simulink model "2014_BEST_default_v5_simulink"  (R2014a)
settings: Solver=FixedStepDiscrete  StartTime=0.0  StopTime=inf  RelTol=1e-3
libraries: vexarmcortexlib x47, simulink x4
settings Model: Creator=shiremat  LastModifiedBy=Caleb Walke
settings DataIOCC: SignalLoggingSaveFormat=ModelDataLogs
settings OptimizationCC: ExpressionDepthLimit=2147483647  OptimizeModelRefInitCode=on  LifeSpan=Inf  MaxStackSize=64
settings DebuggingCC: UnderspecifiedInitializationDetection=Classic  SolverPrmCheckMsg=none  InheritedTsInSrcMsg=none  ParameterPrecisionLossMsg=none  FcnCallInpInsideContextMsg=UseLocalSettings  UnconnectedInputMsg=none  UnconnectedOutputMsg=none  StateNameClashWarn=warning
settings HardwareCC: ProdLargestAtomicInteger=Long  ProdLargestAtomicFloat=Double  ProdIntDivRoundTo=Floor  ProdEndianess=LittleEndian  ProdHWDeviceType=ARM Compatible->ARM Cortex
settings RTWCC: SystemTargetFile=ert.tlc  TemplateMakefile=ert_default_tmf  Description=Embedded Coder  ProcessScript=ert_make_rtw_hook  Toolchain=GNU Tools for VEX ARM Cortex
settings CodeAppCC: IgnoreCustomStorageClasses=off  CustomSymbolStrType=$N$R$M  InternalIdentifier=Classic
settings ERTTargetCC: CodeReplacementLibrary=GCC ARM Cortex-M3  ParMdlRefBuildCompliant=on  CompOptLevelCompliant=on  ConcurrentExecutionCompliant=on  ERTFirstTimeCompliant=on  ModelStepFunctionPrototypeControlCompliant=on  CPPClassGenCompliant=on  InlinedParameterPlacement=Hierarchical

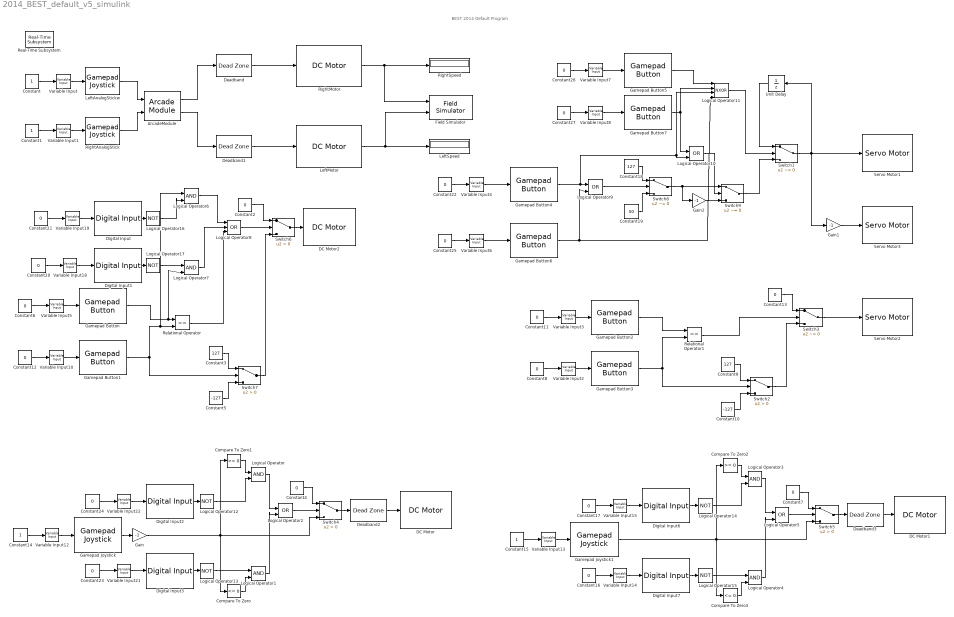
== system 2014_BEST_default_v5_simulink ==
  note: BEST 2014 Default Program
  ArcadeModule : vexarmcortexlib/Utilities/Arcade Module
  Compare To Zero : simulink/Logic and Bit Operations/Compare To Zero  relop=<=  OutDataTypeStr=boolean
  Compare To Zero1 : simulink/Logic and Bit Operations/Compare To Zero  relop=>=  OutDataTypeStr=boolean
  Compare To Zero2 : simulink/Logic and Bit Operations/Compare To Zero  relop=>=  OutDataTypeStr=boolean
  Compare To Zero3 : simulink/Logic and Bit Operations/Compare To Zero  relop=<=  OutDataTypeStr=boolean
  Constant{,1,14..15} (4 alike) : Constant
  Constant10 : Constant  Value=-127
  Constant{6,8,11..13,16..17,20..27} (15 alike) : Constant  Value=0  OutDataTypeStr=boolean
  Constant18 : Constant  Value=127
  Constant19 : Constant  Value=50
  Constant2 : Constant  Value=0
  Constant3 : Constant  Value=127
  Constant4 : Constant  Value=0
  Constant5 : Constant  Value=-127
  Constant7 : Constant  Value=0
  Constant9 : Constant  Value=127
  DC Motor : vexarmcortexlib/DC Motor  motor=5  scaleFactor=1/13.5
  DC Motor1 : vexarmcortexlib/DC Motor  motor=6  scaleFactor=1/13.5
  DC Motor2 : vexarmcortexlib/DC Motor  motor=3  scaleFactor=1/13.5
  Deadband{,1..3} (4 alike) : DeadZone  LowerValue=-4  UpperValue=4  SaturateOnIntegerOverflow=on
  Digital Input : vexarmcortexlib/Digital Input  inChan=1
  Digital Input1 : vexarmcortexlib/Digital Input  inChan=2
  Digital Input2 : vexarmcortexlib/Digital Input  inChan=3
  Digital Input3 : vexarmcortexlib/Digital Input  inChan=4
  Digital Input6 : vexarmcortexlib/Digital Input  inChan=5
  Digital Input7 : vexarmcortexlib/Digital Input  inChan=6
  Field Simulator : vexarmcortexlib/Utilities/Field Simulator  radius=2.5  space=10  range=200
  Gain : Gain  Gain=-1  OutDataTypeStr=Inherit: Inherit via back propagation
  Gain1 : Gain  Gain=-1
  Gain2 : Gain  Gain=-1
  Gamepad Button : vexarmcortexlib/Gamepad Button  joystick=1  chan=5  button56=Down  button78=Right
  Gamepad Button1 : vexarmcortexlib/Gamepad Button  joystick=1  chan=5  button56=Up  button78=Right
  Gamepad Button2 : vexarmcortexlib/Gamepad Button  joystick=1  chan=6  button56=Down  button78=Right
  Gamepad Button3 : vexarmcortexlib/Gamepad Button  joystick=1  chan=6  button56=Up  button78=Right
  Gamepad Button4 : vexarmcortexlib/Gamepad Button  joystick=1  chan=7  button56=Down  button78=Left
  Gamepad Button5 : vexarmcortexlib/Gamepad Button  joystick=1  chan=7  button56=Down  button78=Right
  Gamepad Button6 : vexarmcortexlib/Gamepad Button  joystick=1  chan=7  button56=Down  button78=Down
  Gamepad Button7 : vexarmcortexlib/Gamepad Button  joystick=1  chan=7  button56=Down  button78=Up
  Gamepad Joystick : vexarmcortexlib/Gamepad Joystick  joystick=1  chan=3
  Gamepad Joystick1 : vexarmcortexlib/Gamepad Joystick  joystick=1  chan=4
  LeftAnalogStickw : vexarmcortexlib/Gamepad Joystick  joystick=1  chan=2
  LeftMotor : vexarmcortexlib/DC Motor  motor=9  scaleFactor=1/13.5
  LeftSpeed : Display
  Logical Operator{,1,3..4,6..7} (6 alike) : Logic  IconShape=distinctive  AllPortsSameDT=off  OutDataTypeStr=boolean
  Logical Operator{2,5,9..10} (4 alike) : Logic  Operator=OR  IconShape=distinctive  AllPortsSameDT=off  OutDataTypeStr=boolean
  Logical Operator11 : Logic  Operator=NXOR  Inputs=4  IconShape=distinctive  AllPortsSameDT=off  OutDataTypeStr=boolean
  Logical Operator{12..17} (6 alike) : Logic  Operator=NOT  AllPortsSameDT=off  OutDataTypeStr=boolean
  Logical Operator8 : Logic  Operator=OR  Inputs=3  IconShape=distinctive  AllPortsSameDT=off  OutDataTypeStr=boolean
  Real-Time Subsystem : vexarmcortexlib/Utilities/Real-Time Subsystem  x=1
  Relational Operator : RelationalOperator  Operator===  OutDataTypeStr=boolean
  Relational Operator1 : RelationalOperator  Operator===  OutDataTypeStr=boolean
  RightAnalogStick : vexarmcortexlib/Gamepad Joystick  joystick=1  chan=1
  RightMotor : vexarmcortexlib/DC Motor  motor=2  scaleFactor=1/13.5
  RightSpeed : Display
  Servo Motor1 : vexarmcortexlib/Servo Motor  motor=4  scaleFactor=90/127
  Servo Motor2 : vexarmcortexlib/Servo Motor  motor=7  scaleFactor=90/127
  Servo Motor3 : vexarmcortexlib/Servo Motor  motor=8  scaleFactor=90/127
  Switch{1,3,8..9} (4 alike) : Switch  Criteria=u2 ~= 0
  Switch{2,4..7} (5 alike) : Switch  Criteria=u2 > Threshold
  Unit Delay : UnitDelay  SampleTime=-1
  Variable Input{,1,12..13} (4 alike) : vexarmcortexlib/Utilities/Variable Input  low=-127  gain=0  high=127
  Variable Input{2..8,10,14..15,18..19,21..22} (14 alike) : vexarmcortexlib/Utilities/Variable Input  low=0  gain=0  high=1
  wires:
  LeftMotor/1 -> LeftSpeed/1, Field Simulator/2
  RightMotor/1 -> Field Simulator/1, RightSpeed/1
  Variable Input/1 -> LeftAnalogStickw/1
  Variable Input1/1 -> RightAnalogStick/1
  RightAnalogStick/1 -> ArcadeModule/2
  LeftAnalogStickw/1 -> ArcadeModule/1
  Constant/1 -> Variable Input/1
  Constant1/1 -> Variable Input1/1
  Unit Delay/1 -> Switch1/1
  Switch3/1 -> Servo Motor2/1
  Gamepad Joystick/1 -> Gain/1
  Gain/1 -> Compare To Zero1/1, Compare To Zero/1, Switch4/3
  Digital Input2/1 -> Logical Operator12/1
  Compare To Zero1/1 -> Logical Operator/1
  Digital Input3/1 -> Logical Operator13/1
  Compare To Zero/1 -> Logical Operator1/2
  Logical Operator/1 -> Logical Operator2/1
  Logical Operator1/1 -> Logical Operator2/2
  Logical Operator2/1 -> Switch4/2
  Constant4/1 -> Switch4/1
  Switch4/1 -> Deadband2/1
  Gamepad Joystick1/1 -> Compare To Zero2/1, Compare To Zero3/1, Switch5/3
  Digital Input6/1 -> Logical Operator14/1
  Compare To Zero2/1 -> Logical Operator3/1
  Digital Input7/1 -> Logical Operator15/1
  Compare To Zero3/1 -> Logical Operator4/2
  Logical Operator3/1 -> Logical Operator5/1
  Logical Operator4/1 -> Logical Operator5/2
  Logical Operator5/1 -> Switch5/2
  Constant7/1 -> Switch5/1
  Switch5/1 -> Deadband3/1
  ArcadeModule/1 -> Deadband/1
  ArcadeModule/2 -> Deadband1/1
  Deadband1/1 -> LeftMotor/1
  Deadband/1 -> RightMotor/1
  Constant6/1 -> Variable Input5/1
  Variable Input5/1 -> Gamepad Button/1
  Constant12/1 -> Variable Input10/1
  Variable Input10/1 -> Gamepad Button1/1
  Constant16/1 -> Variable Input14/1
  Variable Input14/1 -> Digital Input7/1
  Constant17/1 -> Variable Input15/1
  Variable Input15/1 -> Digital Input6/1
  Constant20/1 -> Variable Input18/1
  Variable Input18/1 -> Digital Input1/1
  Constant21/1 -> Variable Input19/1
  Variable Input19/1 -> Digital Input/1
  Variable Input12/1 -> Gamepad Joystick/1
  Constant14/1 -> Variable Input12/1
  Variable Input13/1 -> Gamepad Joystick1/1
  Constant15/1 -> Variable Input13/1
  Constant23/1 -> Variable Input21/1
  Variable Input21/1 -> Digital Input3/1
  Constant24/1 -> Variable Input22/1
  Variable Input22/1 -> Digital Input2/1
  Digital Input/1 -> Logical Operator16/1
  Gamepad Button1/1 -> Switch7/2, Logical Operator6/1, Relational Operator/2
  Digital Input1/1 -> Logical Operator17/1
  Gamepad Button/1 -> Logical Operator7/2, Relational Operator/1
  Logical Operator6/1 -> Logical Operator8/1
  Logical Operator8/1 -> Switch6/2
  Constant2/1 -> Switch6/1
  Switch6/1 -> DC Motor2/1
  Logical Operator7/1 -> Logical Operator8/2
  Relational Operator/1 -> Logical Operator8/3
  Constant3/1 -> Switch7/1
  Constant5/1 -> Switch7/3
  Switch7/1 -> Switch6/3
  Constant11/1 -> Variable Input3/1
  Variable Input3/1 -> Gamepad Button2/1
  Constant8/1 -> Variable Input2/1
  Variable Input2/1 -> Gamepad Button3/1
  Gamepad Button2/1 -> Relational Operator1/1
  Gamepad Button3/1 -> Switch2/2, Relational Operator1/2
  Relational Operator1/1 -> Switch3/2
  Constant9/1 -> Switch2/1
  Constant10/1 -> Switch2/3
  Switch2/1 -> Switch3/3
  Constant13/1 -> Switch3/1
  Switch8/1 -> Gain2/1, Switch9/1
  Switch1/1 -> Unit Delay/1, Gain1/1, Servo Motor1/1
  Gain1/1 -> Servo Motor3/1
  Constant18/1 -> Switch8/1
  Constant19/1 -> Switch8/3
  Gain2/1 -> Switch9/3
  Logical Operator9/1 -> Switch8/2
  Gamepad Button4/1 -> Logical Operator11/3, Logical Operator10/2, Logical Operator9/1
  Gamepad Button6/1 -> Logical Operator11/4, Logical Operator9/2
  Gamepad Button7/1 -> Logical Operator11/2, Logical Operator10/1
  Logical Operator10/1 -> Switch9/2
  Switch9/1 -> Switch1/3
  Logical Operator11/1 -> Switch1/2
  Gamepad Button5/1 -> Logical Operator11/1
  Constant22/1 -> Variable Input4/1
  Constant25/1 -> Variable Input6/1
  Constant26/1 -> Variable Input7/1
  Constant27/1 -> Variable Input8/1
  Variable Input7/1 -> Gamepad Button5/1
  Variable Input8/1 -> Gamepad Button7/1
  Variable Input4/1 -> Gamepad Button4/1
  Variable Input6/1 -> Gamepad Button6/1
  Deadband2/1 -> DC Motor/1
  Deadband3/1 -> DC Motor1/1
  Logical Operator12/1 -> Logical Operator/2
  Logical Operator13/1 -> Logical Operator1/1
  Logical Operator14/1 -> Logical Operator3/2
  Logical Operator15/1 -> Logical Operator4/1
  Logical Operator16/1 -> Logical Operator6/2
  Logical Operator17/1 -> Logical Operator7/1
